simulink model "TASK_2"  (R2017a)
settings: Solver=VariableStepAuto  StartTime=0.0  StopTime=10.0  MaxStep=1e-5  RelTol=1e-3
libraries: simulink x1
settings Model: Creator=STUDENT  LastModifiedBy=STUDENT
settings SolverCC: AlgebraicLoopSolver=LineSearch

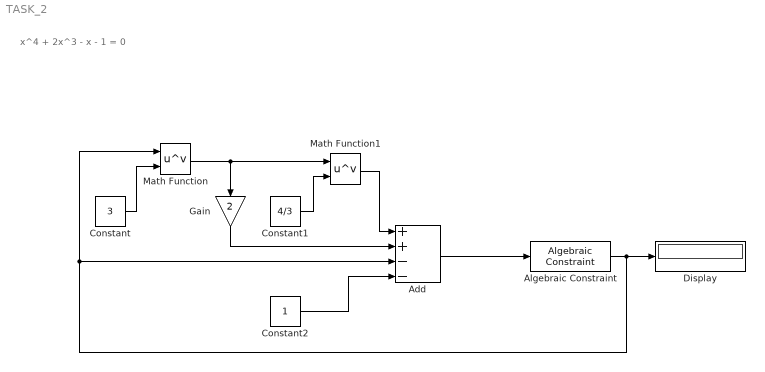
== system TASK_2 ==
  note: x^4 + 2x^3 - x - 1 = 0
  Add : Sum  Inputs=++--
  Algebraic Constraint : simulink/Math Operations/Algebraic Constraint  z0=0
      settings: SourceProductName=Simulink  SourceProductBaseCode=SL
  Constant : Constant  Value=3
  Constant1 : Constant  Value=4/3
  Constant2 : Constant
  Display : Display
  Gain : Gain  Gain=2
  Math Function : Math  Operator=pow  SaturateOnIntegerOverflow=on
  Math Function1 : Math  Operator=pow  SaturateOnIntegerOverflow=on
  wires:
  Constant/1 -> Math Function/2
  Math Function/1 -> Gain/1, Math Function1/1
  Constant1/1 -> Math Function1/2
  Math Function1/1 -> Add/1
  Gain/1 -> Add/2
  Algebraic Constraint/1 -> Display/1, Math Function/1, Add/3
  Constant2/1 -> Add/4
  Add/1 -> Algebraic Constraint/1
